simulink model "IdealSensors"  (R2020b)
settings: Solver=FixedStepAuto  StartTime=0.0  StopTime=10.0  RelTol=1e-3
libraries: aerolibutil x2, dspmathops x1
settings Model: Creator=dbell44  LastModifiedBy=dbell44

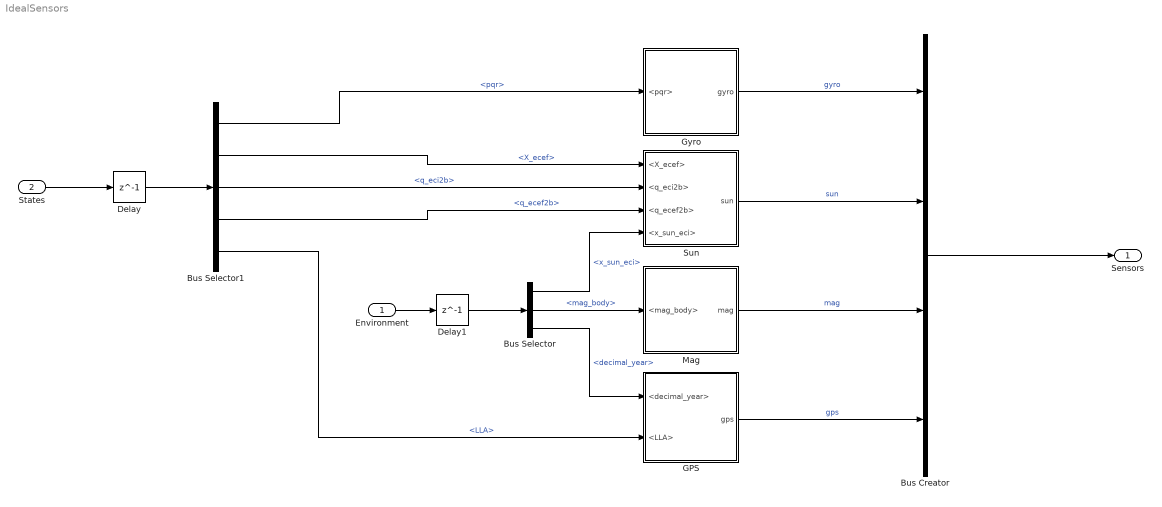
== system IdealSensors ==
  Environment : Inport  OutDataTypeStr=Bus: Environment
  States : Inport  Port=2  OutDataTypeStr=Bus: States
  Bus Creator : BusCreator  Inputs=4  OutDataTypeStr=Bus: Sensors
      settings: InheritFromInputs=off
  Bus Selector : BusSelector  OutputSignals=x_sun_eci,mag_body,decimal_year
  Bus Selector1 : BusSelector  OutputSignals=pqr,X_ecef,q_eci2b,q_ecef2b,LLA
  Delay : Delay  DelayLength=1  InitialCondition=0
  Delay1 : Delay  DelayLength=1  InitialCondition=0
  GPS : Subsystem
  Gyro : Subsystem
  Mag : Subsystem
  Sun : Subsystem
  Sensors : Outport  OutDataTypeStr=Bus: Sensors
  wires:
  Mag/1(mag) -> Bus Creator/3  "mag"
  Sun/1(sun) -> Bus Creator/2  "sun"
  Bus Selector1/3 -> Sun/2(<q_eci2b>)  "<q_eci2b>"
  Bus Selector1/2 -> Sun/1(<X_ecef>)  "<X_ecef>"
  Delay/1 -> Bus Selector1/1
  Bus Selector1/4 -> Sun/3(<q_ecef2b>)  "<q_ecef2b>"
  Bus Selector/2 -> Mag/1(<mag_body>)  "<mag_body>"
  Bus Creator/1 -> Sensors/1
  Bus Selector1/5 -> GPS/2(<LLA>)  "<LLA>"
  Environment/1 -> Delay1/1
  Delay1/1 -> Bus Selector/1
  Bus Selector/3 -> GPS/1(<decimal_year>)  "<decimal_year>"
  States/1 -> Delay/1
  Bus Selector1/1 -> Gyro/1(<pqr>)  "<pqr>"
  Gyro/1(gyro) -> Bus Creator/1  "gyro"
  GPS/1(gps) -> Bus Creator/4  "gps"
  Bus Selector/1 -> Sun/4(<x_sun_eci>)  "<x_sun_eci>"

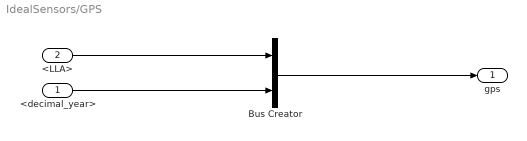
== system IdealSensors/GPS ==
  <decimal_year> : Inport
  <LLA> : Inport  Port=2
  Bus Creator : BusCreator  Inputs=2  OutDataTypeStr=Bus: gnss_data
      settings: InheritFromInputs=off
  gps : Outport  OutDataTypeStr=Bus: gnss_data
  wires:
  <LLA>/1 -> Bus Creator/1
  <decimal_year>/1 -> Bus Creator/2
  Bus Creator/1 -> gps/1

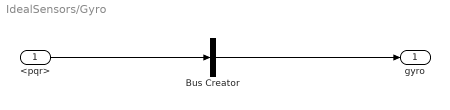
== system IdealSensors/Gyro ==
  <pqr> : Inport
  Bus Creator : BusCreator  Inputs=1  OutDataTypeStr=Bus: gyro_data
      settings: InheritFromInputs=off
  gyro : Outport  OutDataTypeStr=Bus: gyro_data
  wires:
  <pqr>/1 -> Bus Creator/1
  Bus Creator/1 -> gyro/1

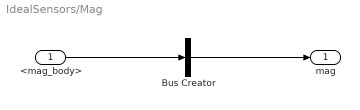
== system IdealSensors/Mag ==
  <mag_body> : Inport
  Bus Creator : BusCreator  Inputs=1  OutDataTypeStr=Bus: mag_data
      settings: InheritFromInputs=off
  mag : Outport  OutDataTypeStr=Bus: mag_data
  wires:
  Bus Creator/1 -> mag/1
  <mag_body>/1 -> Bus Creator/1

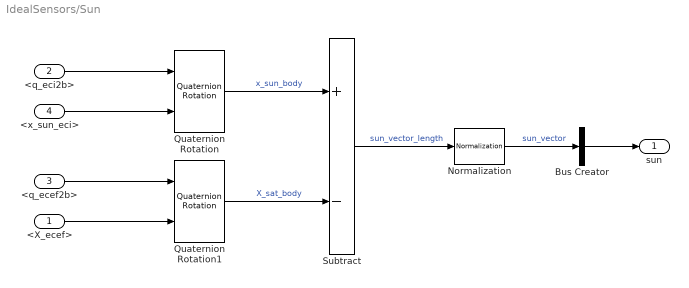
== system IdealSensors/Sun ==
  <X_ecef> : Inport
  <q_eci2b> : Inport  Port=2
  <q_ecef2b> : Inport  Port=3
  <x_sun_eci> : Inport  Port=4
  Bus Creator : BusCreator  Inputs=1  OutDataTypeStr=Bus: sun_data
  Normalization : dspmathops/Normalization  NormType=2-norm  Bias=1e-10  NormOver=Each column  Dimension=1  roundingMode=Floor  overflowMode=off  accumDataTypeStr=Inherit: Same as product output  accumLastDataTypeStr=Inherit: Same as product output  outputDataTypeStr=Inherit: Same as product output  outputMin=[]  outputMax=[]  outputLastDataTypeStr=Inherit: Same as product output
  Quaternion Rotation : aerolibutil/Quaternion Rotation
  Quaternion Rotation1 : aerolibutil/Quaternion Rotation
  Subtract : Sum  Inputs=+-
  sun : Outport  OutDataTypeStr=Bus: sun_data
  wires:
  Bus Creator/1 -> sun/1
  <q_eci2b>/1 -> Quaternion Rotation/1
  <x_sun_eci>/1 -> Quaternion Rotation/2
  Quaternion Rotation/1 -> Subtract/1  "x_sun_body"
  <X_ecef>/1 -> Quaternion Rotation1/2
  <q_ecef2b>/1 -> Quaternion Rotation1/1
  Quaternion Rotation1/1 -> Subtract/2  "X_sat_body"
  Subtract/1 -> Normalization/1  "sun_vector_length"
  Normalization/1 -> Bus Creator/1  "sun_vector"
